simulink model "BasicModel"  (R2019a)
settings: Solver=FixedStepAuto  StartTime=0.0  StopTime=10.0  FixedStep=0.1  RelTol=1e-3
libraries: simulink x8, dspstat3 x1
settings Model: Creator=严龑  LastModifiedBy=严龑

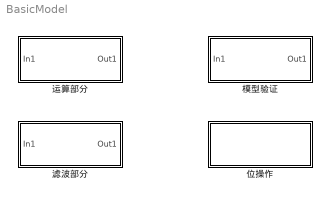
== system BasicModel ==
  位操作 : Subsystem
  模型验证 : Subsystem
  滤波部分 : Subsystem
  运算部分 : Subsystem

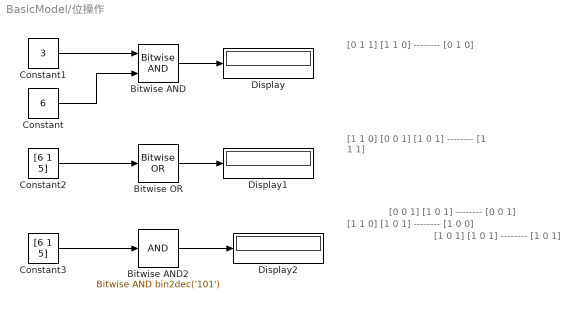
== system BasicModel/位操作 ==
  note: [0 1 1]
      | [1 1 0]
      | --------
      | [0 1 0]
  note: [1 1 0]
      | [0 0 1]
      | [1 0 1]
      | --------
      | [1 1 1]
  note: [1 1 0]
      | [1 0 1]
      | --------
      | [1 0 0]
  note: [0 0 1]
      | [1 0 1]
      | --------
      | [0 0 1]
  note: [1 0 1]
      | [1 0 1]
      | --------
      | [1 0 1]
  Bitwise AND : simulink/Logic and Bit Operations/Bitwise Operator  logicop=AND  UseBitMask=off  NumInputPorts=2  BitMask=bin2dec('11011001')  BitMaskRealWorld=Stored Integer
  Bitwise AND2 : simulink/Logic and Bit Operations/Bitwise Operator  logicop=AND  UseBitMask=on  BitMask=bin2dec('101')  BitMaskRealWorld=Stored Integer
  Bitwise OR : simulink/Logic and Bit Operations/Bitwise Operator  logicop=OR  UseBitMask=off  BitMask=bin2dec('11011001')  BitMaskRealWorld=Stored Integer
  Constant : Constant  Value=6  OutDataTypeStr=uint8
  Constant1 : Constant  Value=3  OutDataTypeStr=uint8
  Constant2 : Constant  Value=[6 1 5]  OutDataTypeStr=uint8
  Constant3 : Constant  Value=[6 1 5]  OutDataTypeStr=uint8
  Display : Display
  Display1 : Display
  Display2 : Display
  wires:
  Constant1/1 -> Bitwise AND/1
  Constant/1 -> Bitwise AND/2
  Bitwise AND/1 -> Display/1
  Constant2/1 -> Bitwise OR/1
  Bitwise OR/1 -> Display1/1
  Constant3/1 -> Bitwise AND2/1
  Bitwise AND2/1 -> Display2/1

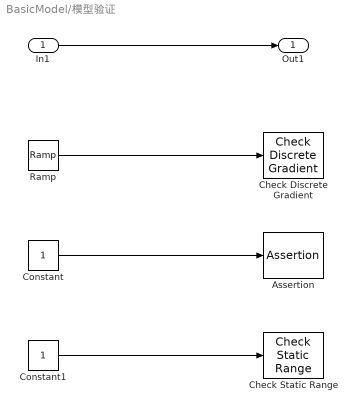
== system BasicModel/模型验证 ==
  In1 : Inport
  Assertion : Assertion
  Check Discrete Gradient : simulink/Model Verification/Check Discrete Gradient  Description=| du / dt | < 1  gradient=1  enabled=on  stopWhenAssertionFail=on  export=off  icon=graphic
      settings: SourceProductName=Simulink  SourceProductBaseCode=SL
  Check Static Range : simulink/Model Verification/Check  Static Range  Description=0 <= u <= 100  max=100  max_included=on  min=0  min_included=on  enabled=on  stopWhenAssertionFail=on  export=off  icon=graphic
      settings: SourceProductName=Simulink  SourceProductBaseCode=SL
  Constant : Constant
  Constant1 : Constant
  Ramp : simulink/Sources/Ramp  slope=1  start=0  InitialOutput=0
  Out1 : Outport
  wires:
  In1/1 -> Out1/1
  Ramp/1 -> Check Discrete Gradient/1
  Constant/1 -> Assertion/1
  Constant1/1 -> Check Static Range/1

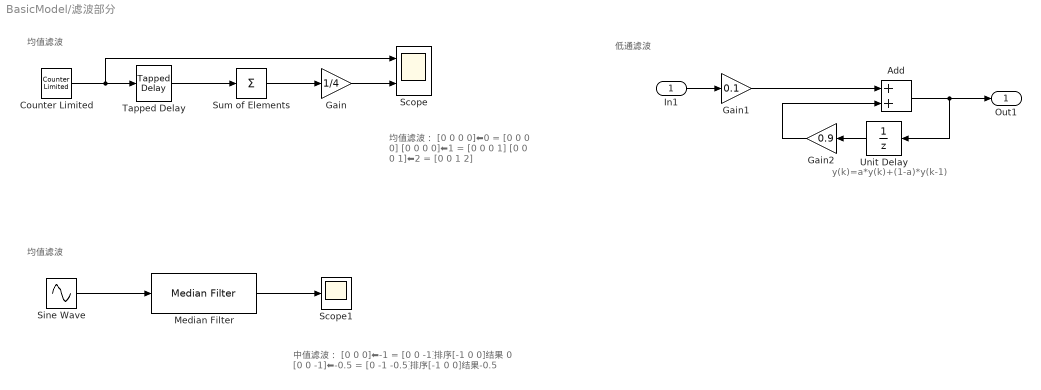
== system BasicModel/滤波部分 ==
  note: y(k)=a*y(k)+(1-a)*y(k-1)
  note: 低通滤波
  note: 均值滤波
  note: 均值滤波：
      | [0 0 0 0]⬅0 = [0 0 0 0]
      | [0 0 0 0]⬅1 = [0 0 0 1]
      | [0 0 0 1]⬅2 = [0 0 1 2]
  note: 均值滤波
  note: 中值滤波：
      | [0 0 0]⬅-1 = [0 0 -1]排序[-1 0 0]结果 0
      | [0 0 -1]⬅-0.5 = [0 -1 -0.5]排序[-1 0 0]结果-0.5
  In1 : Inport
  Add : Sum
  Counter Limited : simulink/Sources/Counter Limited  uplimit=7  tsamp=-1
  Gain : Gain  Gain=1/4
  Gain1 : Gain  Gain=0.1
  Gain2 : Gain  Gain=0.9
  Median Filter : dspstat3/Median Filter  WindowLength=5  SimulateUsing=Interpreted execution
      settings: SourceProductName=DSP System Toolbox  SourceProductBaseCode=DS
  Scope : Scope  NumInputPorts=2
  Scope1 : Scope
  Sine Wave : Sin  SampleTime=0
  Sum of Elements : Sum  Inputs=+
  Tapped Delay : simulink/Discrete/Tapped Delay  vinit=0.0  samptime=-1  NumDelays=4  DelayOrder=Oldest  includeCurrent=off
  Unit Delay : UnitDelay  SampleTime=-1  HasFrameUpgradeWarning=on
  Out1 : Outport
  wires:
  In1/1 -> Gain1/1
  Tapped Delay/1 -> Sum of Elements/1
  Sum of Elements/1 -> Gain/1
  Gain/1 -> Scope/2
  Counter Limited/1 -> Scope/1, Tapped Delay/1
  Sine Wave/1 -> Median Filter/1
  Median Filter/1 -> Scope1/1
  Gain1/1 -> Add/1
  Add/1 -> Unit Delay/1, Out1/1
  Unit Delay/1 -> Gain2/1
  Gain2/1 -> Add/2

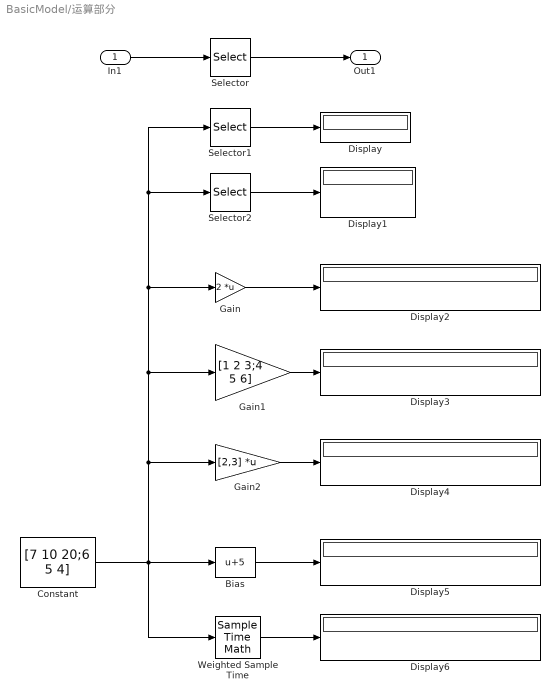
== system BasicModel/运算部分 ==
  In1 : Inport
  Bias : Bias  Bias=5
  Constant : Constant  Value=[7 10 20;6 5 4]
  Display{,1..6} (7 alike) : Display
  Gain : Gain  Gain=2  Multiplication=Matrix(K*u)
  Gain1 : Gain  Gain=[1 2 3;4 5 6]
  Gain2 : Gain  Gain=[2,3]  Multiplication=Matrix(K*u)
  Selector : Selector  InputPortWidth=3  IndexOptions=Index vector (dialog)  Indices=[1 3]  OutputSizes=1
  Selector1 : Selector  NumberOfDimensions=2  InputPortWidth=3  IndexOptions=Index vector (dialog),Index vector (dialog)  Indices=2,1  OutputSizes=1,1
  Selector2 : Selector  NumberOfDimensions=2  InputPortWidth=3  IndexOptions=Index vector (dialog),Index vector (dialog)  Indices=[1 2],2  OutputSizes=1,1
  Weighted Sample Time : SampleTimeMath
  Out1 : Outport
  wires:
  In1/1 -> Selector/1
  Selector/1 -> Out1/1
  Selector1/1 -> Display/1
  Selector2/1 -> Display1/1
  Gain/1 -> Display2/1
  Constant/1 -> Selector2/1, Selector1/1, Gain/1, Gain1/1, Gain2/1, Bias/1, Weighted Sample Time/1
  Gain1/1 -> Display3/1
  Gain2/1 -> Display4/1
  Bias/1 -> Display5/1
  Weighted Sample Time/1 -> Display6/1
